simulink model "es2a_sim"  (Simulink 7.9)
settings: Solver=ode45  StartTime=0.0  StopTime=10.0  RelTol=1e-3
values from neighbouring files (symbols this model uses):
  A = [-1.9 -1.2 -1.9;-1.9 -2.2 -0.9;2.1 1.8 1.1]    [es2a.m]
  B = [0.4 0.4 -0.6]'    [es2a.m]
  C = [0 0 1]    [es2a.m]
  ueq = 3    [es2a.m]
  x0 = [0 0 0]    [es2a.m]
settings Model: Creator=claudio  LastModifiedBy=patrizio
settings OptimizationCC: InitFltsAndDblsToZero=on
settings DebuggingCC: FcnCallInpInsideContextMsg=Use local settings  StrictBusMsg=Warning
settings GRTTargetCC: CombineOutputUpdateFcns=off  GRTInterface=on

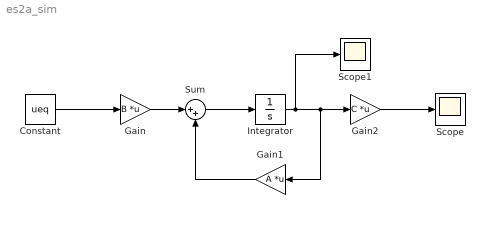
== system es2a_sim ==
  Constant : Constant  Value=ueq
  Gain : Gain  Gain=B  Multiplication=Matrix(K*u)
  Gain1 : Gain  Gain=A  Multiplication=Matrix(K*u)
  Gain2 : Gain  Gain=C  Multiplication=Matrix(K*u)
  Integrator : Integrator  InitialCondition=x0
  Scope : Scope
  Scope1 : Scope
  Sum : Sum  Inputs=|++
  wires:
  Constant/1 -> Gain/1
  Gain/1 -> Sum/1
  Gain1/1 -> Sum/2
  Sum/1 -> Integrator/1
  Integrator/1 -> Gain2/1, Gain1/1, Scope1/1
  Gain2/1 -> Scope/1
